simulink model "twothree"  (R2014a)
settings: Solver=ode45  StartTime=0.0  StopTime=15  MaxStep=0.001  MinStep=0.0001  RelTol=1e-3
libraries: simulink x1
settings Model: Creator=trigg  LastModifiedBy=trigg

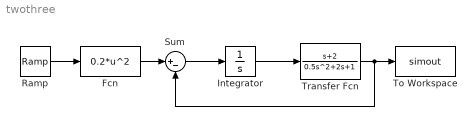
== system twothree ==
  Fcn : Fcn  Expr=0.2*u^2
  Integrator : Integrator  InitialCondition=1
  Ramp : simulink/Sources/Ramp  slope=1  start=0  X0=0
  Sum : Sum  Inputs=|+-
  To Workspace : ToWorkspace  VariableName=simout  SaveFormat=Timeseries  SampleTime=-1
  Transfer Fcn : TransferFcn  Numerator=[1 2]  Denominator=[0.5 2 1]
  wires:
  Fcn/1 -> Sum/1
  Sum/1 -> Integrator/1
  Integrator/1 -> Transfer Fcn/1
  Transfer Fcn/1 -> To Workspace/1, Sum/2
  Ramp/1 -> Fcn/1
